simulink model "NN_MPC"  (R2018a)
settings: Solver=FixedStepAuto  SolverName=VariableStepAuto  StartTime=0.0  StopTime=40  FixedStep=0.01  RelTol=1e-3
values from neighbouring files (symbols this model uses):
  a = 0.95    [Params.mat]    (also in R_neural_function.m = 2 ./ (1 + exp(-2*n)) - 1; neural_Nc.m = 2 ./ (1 + exp(-2*n)) - 1; neural_Np.m = 2 ./ (1 + exp(-2*n)) - 1; neural_Qy.m = 2 ./ (1 + exp(-2*n)) - 1)
  Cf = 19000    [Params.mat]
  Cr = 33000    [Params.mat]
  deltau_max = 0.261799387799    [Params.mat]
  deltau_min = -0.261799387799    [Params.mat]
  dt = 0.1    [Params.mat]
  Iz = 2875    [Params.mat]
  lf = 1.2    [Params.mat]
  lr = 1.6    [Params.mat]
  m = 1575    [Params.mat]
  N = 10    [Params.mat]
  Nc = 5    [Params.mat]
  Np = 35    [Params.mat]
  Q = 5    [Params.mat]    (also in R_neural_function.m = 0; neural_Nc.m = 0; neural_Np.m = 0; neural_Qy.m = 0)
  R = 0.1    [Params.mat]
  u_max = 0.523598775598    [Params.mat]
  u_min = -0.523598775598    [Params.mat]
  y_max = 200    [Params.mat]
  y_min = -200    [Params.mat]
undefined symbols (not defined in the file or in its folder): neural_Nc, neural_Np, neural_Qy, neural_R, sigbuilder_block
libraries: autolibutils x8, autolibshared x6, vehdynlibviscommon x2, simulink x2
(part 4 of 4)

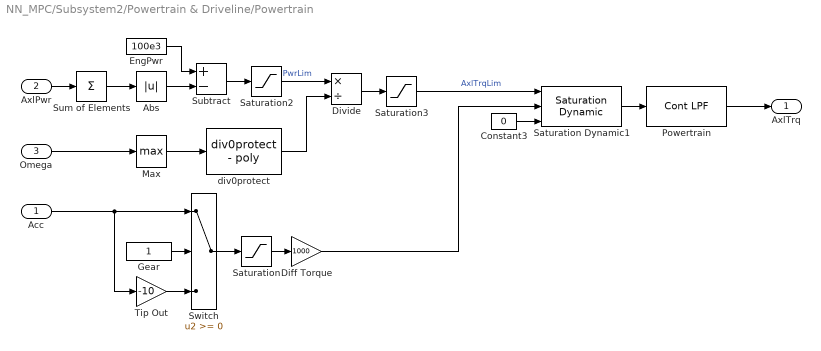
== system NN_MPC/Subsystem2/Powertrain & Driveline/Powertrain ==
  Acc : Inport
  AxlPwr : Inport  Port=2
  Omega : Inport  Port=3
  Abs : Abs  ZeroCross=off
  Constant3 : Constant  Value=0
  Diff Torque : Gain  Gain=1000
  Divide : Product  Inputs=*/
  EngPwr : Constant  Value=100e3
  Gear : Constant  SampleTime=-1
  Max : MinMax  Function=max  ZeroCross=off
  Powertrain : autolibutils/Cont LPF  wc=4*pi*2  AbsoluteTolerance=auto  aMode=2
  Saturation : Saturate  UpperLimit=inf  LowerLimit=0  ZeroCross=off
  Saturation Dynamic1 : simulink/Discontinuities/Saturation Dynamic  OutMin=[]  OutMax=[]  OutDataTypeStr=Inherit: Same as second input  OutDataType=fixdt(1, 16)  OutScaling=2^-10  DoSatur=off
  Saturation2 : Saturate  UpperLimit=inf  LowerLimit=100  ZeroCross=off
  Saturation3 : Saturate  UpperLimit=1000  LowerLimit=0  ZeroCross=off
  Subtract : Sum  Inputs=+-
  Sum of Elements : Sum  Inputs=+
  Switch : Switch  ZeroCross=off
  Tip Out : Gain  Gain=-10
  div0protect : autolibutils/div0protect - poly  thresh=1  ZeroCross1=on  aMode=2
  AxlTrq : Outport  VectorParamsAs1DForOutWhenUnconnected=off
  wires:
  Max/1 -> div0protect/1
  Saturation3/1 -> Saturation Dynamic1/1  "AxlTrqLim"
  AxlPwr/1 -> Sum of Elements/1
  EngPwr/1 -> Subtract/1
  Saturation2/1 -> Divide/1  "PwrLim"
  Subtract/1 -> Saturation2/1
  Omega/1 -> Max/1
  div0protect/1 -> Divide/2
  Divide/1 -> Saturation3/1
  Abs/1 -> Subtract/2
  Sum of Elements/1 -> Abs/1
  Constant3/1 -> Saturation Dynamic1/3
  Tip Out/1 -> Switch/3
  Saturation Dynamic1/1 -> Powertrain/1
  Gear/1 -> Switch/2
  Diff Torque/1 -> Saturation Dynamic1/2
  Saturation/1 -> Diff Torque/1
  Acc/1 -> Switch/1, Tip Out/1
  Switch/1 -> Saturation/1
  Powertrain/1 -> AxlTrq/1

== system NN_MPC/Subsystem1/Powertrain & Driveline1/Driveline/AWD ==
  TPowertrain : Inport
  AWD : Gain  Gain=[1;1;1;1]./2
  TAxles : Outport  VectorParamsAs1DForOutWhenUnconnected=off
  wires:
  TPowertrain/1 -> AWD/1
  AWD/1 -> TAxles/1

== system NN_MPC/Subsystem1/Powertrain & Driveline1/Driveline/FWD ==
  TPowertrain : Inport
  FWD : Gain  Gain=[1;1;0;0]
  TAxles : Outport  VectorParamsAs1DForOutWhenUnconnected=off
  wires:
  FWD/1 -> TAxles/1
  TPowertrain/1 -> FWD/1

== system NN_MPC/Subsystem1/Powertrain & Driveline1/Driveline/RWD ==
  TPowertrain : Inport
  RWD : Gain  Gain=[0;0;1;1]
  TAxles : Outport  VectorParamsAs1DForOutWhenUnconnected=off
  wires:
  TPowertrain/1 -> RWD/1
  RWD/1 -> TAxles/1

== system NN_MPC/Subsystem2/Powertrain & Driveline/Driveline/AWD ==
  TPowertrain : Inport
  AWD : Gain  Gain=[1;1;1;1]./2
  TAxles : Outport  VectorParamsAs1DForOutWhenUnconnected=off
  wires:
  TPowertrain/1 -> AWD/1
  AWD/1 -> TAxles/1

== system NN_MPC/Subsystem2/Powertrain & Driveline/Driveline/FWD ==
  TPowertrain : Inport
  FWD : Gain  Gain=[1;1;0;0]
  TAxles : Outport  VectorParamsAs1DForOutWhenUnconnected=off
  wires:
  FWD/1 -> TAxles/1
  TPowertrain/1 -> FWD/1

== system NN_MPC/Subsystem2/Powertrain & Driveline/Driveline/RWD ==
  TPowertrain : Inport
  RWD : Gain  Gain=[0;0;1;1]
  TAxles : Outport  VectorParamsAs1DForOutWhenUnconnected=off
  wires:
  TPowertrain/1 -> RWD/1
  RWD/1 -> TAxles/1

== matlab function NN_MPC/Subsystem1/MPC1 ==
  settings: updateMethod=DISCRETE
  data: u output; Vx input; u input; y input; r input; m input; Iz input; lf input; lr input; Cf input; Cr input; dt input; a input; N input; Nc input; Np input; Qy input; R input; u_min input; u_max input; deltau_min input; deltau_max input; y_min input; y_max input; xm input
%%%%%%%%%%%%%%%%%%%%%%%%%%%%%%%%%%%%%%%%%%%%%%%%%%%%%%%%%%%%%%%%%%%%%%%%%%%
% Author: Yassine Kebbati
% Date: 10/03/2021
% Control DMPC-Autonomous_Driving
%%%%%%%%%%%%%%%%%%%%%%%%%%%%%%%%%%%%%%%%%%%%%%%%%%%%%%%%%%%%%%%%%%%%%%%%%%%
function u = fcn(Vx, u,y,r,m,Iz,lf,lr,Cf,Cr,dt,a,N,Nc,Np,Qy,R,u_min,u_max,deltau_min,deltau_max,y_min,y_max,xm)

tic;

coder.extrinsic('c2dm')
%coder.extrinsic(function)

%load('new_trajectory.mat')


% Model identification

% m = 1575;
% Iz = 2875;
% lf = 1.2;
% lr = 1.6;
% Cf = 19000;
% Cr = 33000;


%state vector  [y_dot phi phi_dot y]
Ac = [-(2*Cf+2*Cr)/m/Vx, 0, -Vx-(2*Cf*lf-2*Cr*lr)/m/Vx, 0;
     0, 0, 1, 0;
     -(2*Cf*lf-2*Cr*lr)/Iz/Vx, 0, -(2*Cf*lf^2+2*Cr*lr^2)/Iz/Vx, 0;
     1, Vx, 0, 0];
Bc = [2*Cf/m 0 2*Cf*lf/Iz 0]';   
Cc = [0 0 0 1];
%C2 = [0 0 0 1; 0 1 0 0];
Dc = zeros(1,1);

%dt=0.1;
[Ad, Bd, Cd, Dd]=c2dm(Ac,Bc,Cc,Dc,dt,'zoh');
% tic
% Make the augmented state-space model
n1 = 0;
m1 = 0;
n_in = 0;

[m1, n1] = size(Cd);
[n1, n_in] = size(Bd);
A = eye(n1+m1, n1+m1);
A(1:n1, 1:n1) = Ad;
A(n1+1:n1+m1,1:n1) = Cd*Ad;
B = zeros(n1+m1, n_in);
B(1:n1,:) = Bd;
B(n1+1:n1+m1,:) = Cd*Bd;
C = zeros(m1, n1+m1);
C(:, n1+1:n1+m1) = eye(m1, m1);
D = Dd;


% a=0.5;
% Nc=5;
% N=5; %you can increase N
% Np=25;

%obtain constraints data matrices

[M1,Lzerot]=Mdu(a,N,1,Nc);
M0=Mu(a,N,1,Nc);

%initial conditions for closed-loop simulation using constrained control
%specify the limits for ?u and u

%xm=zeros(n1,1);
% persistent xm;
% if isempty(xm)
%   xm=zeros(n1,1);
% end


persistent xm_old
if isempty(xm_old)
  %xm_old=[0; 0; 0; 37];
  xm_old=zeros(4,1);
end


persistent Xf
if isempty(Xf)
  Xf=[xm; y-r];
end


Xf=[xm-xm_old;y-r];
%end
xm_old=xm;

%specify constraints limits

% u_min=-pi/6;
% u_max=pi/6;
% deltau_min=-pi/12;
% deltau_max=pi/12;
% 
%  y_min=-2;
%  y_max=6;
y_bar_min=y_min-r;
y_bar_max=y_max-r;


%up=0.0;
up=u;

% C2 = [0 0 0 1; 0 1 0 0];
% Cc = [0 0 0 1];
% Generate matrices required for the predictive control cost function J

% Q=C'*C;
% R=0.0001;
Q=[0,0,0,0,0;0,0,0,0,0;0,0,0,0,0;0,0,0,0,0;0,0,0,0,Qy];


%for kk=1:N_sim-1;
% Continuous-time model

% Ac = [-(2*Cf+2*Cr)/m, 0, -Vx-(2*Cf*lf-2*Cr*lr)/(m*Vx), 0;
%      0, 0, 1, 0;
%      -(2*Cf*lf-2*Cr*lr)/Iz/Vx, 0, -(2*Cf*lf^2+2*Cr*lr^2)/Iz/Vx, 0;
%      1, Vx, 0, 0];
% Bc = [2*Cf/m 0 2*Cf*lf/Iz 0]';   
% Cc = [0 0 0 1];
% C2 = [0 0 0 1; 0 1 0 0];
% Dc = zeros(1,1);

% Minimal realisation

% [num,den] = ss2tf(Ac,Bc,Cc,Dc);
% Gs = tf(num,den);
% 
% Gsmin=ss(Gs,'min');
% [Am,Bm,Cm,Dm]=ssdata(Gsmin);

% Discrete-time model

% dt=0.1;
% [Ad, Bd, Cd, Dd]=c2dm(Ac,Bc,Cc,Dc,dt,'zoh');

% Make the augmented state-space model

% [m1, n1] = size(Cd);
% [n1, n_in] = size(Bd);
% A = eye(n1+m1, n1+m1);
% A(1:n1, 1:n1) = Ad;
% A(n1+1:n1+m1,1:n1) = Cd*Ad;
% B = zeros(n1+m1, n_in);
% B(1:n1,:) = Bd;
% B(n1+1:n1+m1,:) = Cd*Bd;
% C = zeros(m1, n1+m1);
% C(:, n1+1:n1+m1) = eye(m1, m1);
% D = Dd;



[Phi,F]=mpcgain(Ad,Bd,Cd,N,Np);
[Omega,Psi]=dmpc(A,B,a,N,Np,Q,R);







%% constrains on U first
 M=[M0;-M0;M1;-M1;Phi(1:Nc,1)*Lzerot;-Phi(1:Nc,1)*Lzerot];


%closed-loop simulation performed recursively
%optimal control is also found recursively

%% constrains on u first
gamma=[(u_max-up)*ones(Nc,1);(-u_min+up)*ones(Nc,1);...
    deltau_max*ones(Nc,1);-deltau_min*ones(Nc,1);...
    y_bar_max-F(1:Nc,:)*Xf;-y_bar_min+F(1:Nc,:)*Xf];

eta=QPhild(Omega,Psi*Xf,M,gamma);

deltau=Lzerot*eta;
if (deltau>deltau_max) deltau=deltau_max;end
if (deltau<deltau_min) deltau=deltau_min;end
u=u+deltau;
if (u>u_max) deltau=u_max-up; u=u_max; end
if (u<u_min) deltau=u_min-up; u=u_min; end


%deltau1(1,kk)=deltau; %save data
%u1(1,kk)=u; %save data
%y1(:,kk)=y; %save data

%%%%
%plant simulation
%%%%%%


% xm=Ad*xm+Bd*u; % calculate xm(k+1)
% y=Cd*xm; %calculate y(k+1)
% y2=C2*xm;
% y3(1,kk)=y2(2,1);
% Xf=[xm-xm_old;y-r(1,kk)];
% y_bar_min=y_min-r(1,kk);
% y_bar_max=y_max-r(1,kk);

%timeElapsed = toc

== matlab function NN_MPC/Subsystem2/MPC ==
  settings: updateMethod=DISCRETE
  data: u output; Vx input; u input; y input; r input; m input; Iz input; lf input; lr input; Cf input; Cr input; dt input; a input; N input; Nc input; Np input; Qy input; R input; u_min input; u_max input; deltau_min input; deltau_max input; y_min input; y_max input; xm input
%%%%%%%%%%%%%%%%%%%%%%%%%%%%%%%%%%%%%%%%%%%%%%%%%%%%%%%%%%%%%%%%%%%%%%%%%%%
% Author: Yassine Kebbati
% Date: 10/03/2021
% Control DMPC-Autonomous_Driving
%%%%%%%%%%%%%%%%%%%%%%%%%%%%%%%%%%%%%%%%%%%%%%%%%%%%%%%%%%%%%%%%%%%%%%%%%%%
function u = fcn(Vx, u,y,r,m,Iz,lf,lr,Cf,Cr,dt,a,N,Nc,Np,Qy,R,u_min,u_max,deltau_min,deltau_max,y_min,y_max,xm)

tic;

coder.extrinsic('c2dm')
%coder.extrinsic(function)

%load('new_trajectory.mat')


% Model identification

% m = 1575;
% Iz = 2875;
% lf = 1.2;
% lr = 1.6;
% Cf = 19000;
% Cr = 33000;


%state vector  [y_dot phi phi_dot y]
Ac = [-(2*Cf+2*Cr)/m/Vx, 0, -Vx-(2*Cf*lf-2*Cr*lr)/m/Vx, 0;
     0, 0, 1, 0;
     -(2*Cf*lf-2*Cr*lr)/Iz/Vx, 0, -(2*Cf*lf^2+2*Cr*lr^2)/Iz/Vx, 0;
     1, Vx, 0, 0];
Bc = [2*Cf/m 0 2*Cf*lf/Iz 0]';   
Cc = [0 0 0 1];
%C2 = [0 0 0 1; 0 1 0 0];
Dc = zeros(1,1);

%dt=0.1;
[Ad, Bd, Cd, Dd]=c2dm(Ac,Bc,Cc,Dc,dt,'zoh');
% tic
% Make the augmented state-space model
n1 = 0;
m1 = 0;
n_in = 0;

[m1, n1] = size(Cd);
[n1, n_in] = size(Bd);
A = eye(n1+m1, n1+m1);
A(1:n1, 1:n1) = Ad;
A(n1+1:n1+m1,1:n1) = Cd*Ad;
B = zeros(n1+m1, n_in);
B(1:n1,:) = Bd;
B(n1+1:n1+m1,:) = Cd*Bd;
C = zeros(m1, n1+m1);
C(:, n1+1:n1+m1) = eye(m1, m1);
D = Dd;


% a=0.5;
% Nc=5;
% N=5; %you can increase N
% Np=25;

%obtain constraints data matrices

[M1,Lzerot]=Mdu(a,N,1,Nc);
M0=Mu(a,N,1,Nc);

%initial conditions for closed-loop simulation using constrained control
%specify the limits for ?u and u

%xm=zeros(n1,1);
% persistent xm;
% if isempty(xm)
%   xm=zeros(n1,1);
% end


persistent xm_old
if isempty(xm_old)
  %xm_old=[0; 0; 0; 37];
  xm_old=zeros(4,1);
end


persistent Xf
if isempty(Xf)
  Xf=[xm; y-r];
end


Xf=[xm-xm_old;y-r];
%end
xm_old=xm;

%specify constraints limits

% u_min=-pi/6;
% u_max=pi/6;
% deltau_min=-pi/12;
% deltau_max=pi/12;
% 
%  y_min=-2;
%  y_max=6;
y_bar_min=y_min-r;
y_bar_max=y_max-r;


%up=0.0;
up=u;

% C2 = [0 0 0 1; 0 1 0 0];
% Cc = [0 0 0 1];
% Generate matrices required for the predictive control cost function J

% Q=C'*C;
% R=0.0001;
Q=[0,0,0,0,0;0,0,0,0,0;0,0,0,0,0;0,0,0,0,0;0,0,0,0,Qy];


%for kk=1:N_sim-1;
% Continuous-time model

% Ac = [-(2*Cf+2*Cr)/m, 0, -Vx-(2*Cf*lf-2*Cr*lr)/(m*Vx), 0;
%      0, 0, 1, 0;
%      -(2*Cf*lf-2*Cr*lr)/Iz/Vx, 0, -(2*Cf*lf^2+2*Cr*lr^2)/Iz/Vx, 0;
%      1, Vx, 0, 0];
% Bc = [2*Cf/m 0 2*Cf*lf/Iz 0]';   
% Cc = [0 0 0 1];
% C2 = [0 0 0 1; 0 1 0 0];
% Dc = zeros(1,1);

% Minimal realisation

% [num,den] = ss2tf(Ac,Bc,Cc,Dc);
% Gs = tf(num,den);
% 
% Gsmin=ss(Gs,'min');
% [Am,Bm,Cm,Dm]=ssdata(Gsmin);

% Discrete-time model

% dt=0.1;
% [Ad, Bd, Cd, Dd]=c2dm(Ac,Bc,Cc,Dc,dt,'zoh');

% Make the augmented state-space model

% [m1, n1] = size(Cd);
% [n1, n_in] = size(Bd);
% A = eye(n1+m1, n1+m1);
% A(1:n1, 1:n1) = Ad;
% A(n1+1:n1+m1,1:n1) = Cd*Ad;
% B = zeros(n1+m1, n_in);
% B(1:n1,:) = Bd;
% B(n1+1:n1+m1,:) = Cd*Bd;
% C = zeros(m1, n1+m1);
% C(:, n1+1:n1+m1) = eye(m1, m1);
% D = Dd;



[Phi,F]=mpcgain(Ad,Bd,Cd,N,Np);
[Omega,Psi]=dmpc(A,B,a,N,Np,Q,R);







%% constrains on U first
 M=[M0;-M0;M1;-M1;Phi(1:Nc,1)*Lzerot;-Phi(1:Nc,1)*Lzerot];


%closed-loop simulation performed recursively
%optimal control is also found recursively

%% constrains on u first
gamma=[(u_max-up)*ones(Nc,1);(-u_min+up)*ones(Nc,1);...
    deltau_max*ones(Nc,1);-deltau_min*ones(Nc,1);...
    y_bar_max-F(1:Nc,:)*Xf;-y_bar_min+F(1:Nc,:)*Xf];

eta=QPhild(Omega,Psi*Xf,M,gamma);

deltau=Lzerot*eta;
if (deltau>deltau_max) deltau=deltau_max;end
if (deltau<deltau_min) deltau=deltau_min;end
u=u+deltau;
if (u>u_max) deltau=u_max-up; u=u_max; end
if (u<u_min) deltau=u_min-up; u=u_min; end


%deltau1(1,kk)=deltau; %save data
%u1(1,kk)=u; %save data
%y1(:,kk)=y; %save data

%%%%
%plant simulation
%%%%%%


% xm=Ad*xm+Bd*u; % calculate xm(k+1)
% y=Cd*xm; %calculate y(k+1)
% y2=C2*xm;
% y3(1,kk)=y2(2,1);
% Xf=[xm-xm_old;y-r(1,kk)];
% y_bar_min=y_min-r(1,kk);
% y_bar_max=y_max-r(1,kk);

%timeElapsed = toc

== matlab function NN_MPC/Neural Network/MATLAB Function1 ==
  data: nc input; Nc output
%%%%%%%%%%%%%%%%%%%%%%%%%%%%%%%%%%%%%%%%%%%%%%%%%%%%%%%%%%%%%%%%%%%%%%%%%%%
% Author: Yassine Kebbati
% Date: 10/04/2021
% Control NNMPC-Autonomous_Driving
%%%%%%%%%%%%%%%%%%%%%%%%%%%%%%%%%%%%%%%%%%%%%%%%%%%%%%%%%%%%%%%%%%%%%%%%%%%
function Nc = fcn(nc)

nc = round(nc);
if nc<5
    nc = 5;
end
Nc=nc;

== matlab function NN_MPC/Neural Network/MATLAB Function2 ==
  data: nc input; np input; Np output
%%%%%%%%%%%%%%%%%%%%%%%%%%%%%%%%%%%%%%%%%%%%%%%%%%%%%%%%%%%%%%%%%%%%%%%%%%%
% Author: Yassine Kebbati
% Date: 10/04/2021
% Control NNMPC-Autonomous_Driving
%%%%%%%%%%%%%%%%%%%%%%%%%%%%%%%%%%%%%%%%%%%%%%%%%%%%%%%%%%%%%%%%%%%%%%%%%%%
function Np = fcn(nc,np)

np = round(np);
if np<9
    np = 9;
end
if np < nc
    np = nc + 3;
end
Np=np;

== matlab function NN_MPC/Neural Network/MATLAB Function3 ==
  data: qy input; Qy output
%%%%%%%%%%%%%%%%%%%%%%%%%%%%%%%%%%%%%%%%%%%%%%%%%%%%%%%%%%%%%%%%%%%%%%%%%%%
% Author: Yassine Kebbati
% Date: 10/04/2021
% Control NNMPC-Autonomous_Driving
%%%%%%%%%%%%%%%%%%%%%%%%%%%%%%%%%%%%%%%%%%%%%%%%%%%%%%%%%%%%%%%%%%%%%%%%%%%
function Qy = fcn(qy)

if qy<0.75
    qy = 0.75;
end
if qy >10
qy=10;
end

Qy=qy;

== matlab function NN_MPC/Neural Network/MATLAB Function4 ==
  data: r input; R output
%%%%%%%%%%%%%%%%%%%%%%%%%%%%%%%%%%%%%%%%%%%%%%%%%%%%%%%%%%%%%%%%%%%%%%%%%%%
% Author: Yassine Kebbati
% Date: 10/04/2021
% Control NNMPC-Autonomous_Driving
%%%%%%%%%%%%%%%%%%%%%%%%%%%%%%%%%%%%%%%%%%%%%%%%%%%%%%%%%%%%%%%%%%%%%%%%%%%
function R = fcn(r)

if r<0.01
    r = 0.01;
end
if r>0.5
r=0.5;
end

R=r;
